simulink model "EcoSIM3_P2_C2_WIP"  (R2014b)
settings: Solver=ode1  SolverMode=SingleTasking  StartTime=0.0  StopTime=4  FixedStep=0.01  RelTol=1e-3
PostLoadFcn:
  | %, if any(exist('dsrtsu_mdlpostloadfcn', 'file') == [2, 3, 6]), try dsrtsu_mdlpostloadfcn('Execute', bdroot); catch fprintf('Error in PostLoadFcn (dsrtsu_mdlpostloadfcn) for model "%s":\n %s\n', bdroot, lasterr); end, end,
InitFcn:
  | tic
  | %Startup_EcoSIM
undefined symbols (not defined in the file or in its folder): canChannel, Controls, DriveCycles, Driver, EM_EFF_MAP, EM_PwrLoss_MAP, EngPwr, EngSpd, EngTrq, Glbl, Overwritten_Mode, Plants, Power, sigbuilder_block, Torque, Trialmap, Veh_Dynamics
libraries: simulink x135, canmsglib x113, fl_lib x104, canlib x89, nesl_utility x56, sdl_lib x29, dspsigops x6, dspswit3 x5, dspstat3 x2, commnoisgen2 x1, dspfdesign x1
(part 1 of 21)
settings Model: DSRTSU_INTERNAL_RTI_VER=450  DSRTSU_INTERNAL_RTI_TYPE=rti1006  RTICANMMDATA=struct('GeneralSetupData',struct('modelroot','C:\Users\EcoCAR_HIL\Documents\Khanna\EcoSIM3_P1_0_PHEV_dynamic_RTI','generalsettings',struct('filesettings',struct('destfolder',struct('Name','RTICANMM_FILES','Check',1),'buildfolder',struct('Name','.','Check',1),'AbsDestfolder',struct('Name','C:\Users\EcoCAR_HIL\Documents\Khanna\EcoSIM3_P1_0_PHEV_dynamic_RTI\RTICANMM_FILES'),'AbsBuildfolder',struct('Name','C:\Users\EcoCAR_HIL\Documents\Khanna\EcoSIM3_P1_0_PHEV_dynamic_RTI'))),'options',struct('addpaths',1,'rmpaths',1,'addtrcexclusion',logical(1),'cannavigator',struct('checkmonitoring',0),'show_usrtrc',0,'use_usrtrc',0),'advanced',struct('options',[1 1 1 1 1 1 1 1 1 1 1 1 1 1 1 1 1 1 1 1 1 1 1 1 1 1 1 1 1 1 1 1 1 1 1 1 1 1 1 1 1 1 1 1 1 1 1 1 1 1 1 1 1 1 1 1 1 1 1 1 1 1 1 1 1 1 1 1 1 1 1 1 1 1 1 1 1 1 1 1 1 1 1 1 1 1 1 1 1 1 1 1 1 1 1 1 1 1 1 1]),'MPSetup',{{}},'modelname','EcoSIM3_P1_0_PHEV_2014b_with_inertia','block','EcoSIM3_P1_0_PHEV_2014b_with_inertia'))  DSRTSU_INTERNAL_RTIFPGA=40  CovPath=GCM/ProcessMode  CovHTMLOptions=-sRT=1 -sVT=0 -aTS=1 -bRG=1 -bTC=1 -hTR=0 -nFC=0 -scm=1 -bcm=1 -xEv=0  Creator=Arjun  LastModifiedBy=Aditya
settings ConfigSet: Description=This configuration is meant for HIL simulations. During HIL simulations, the model should use dSPACE's rti1006 to generate code.
settings DataIOCC: InspectSignalLogs=on
settings OptimizationCC: BlockReduction=off
settings DebuggingCC: UnderspecifiedInitializationDetection=Classic  MergeDetectMultiDrivingBlocksExec=none  MultiTaskCondExecSysMsg=warning
settings HardwareCC: ProdIntDivRoundTo=Zero  ProdEndianess=LittleEndian  ProdHWDeviceType=Generic->Custom  TargetIntDivRoundTo=Zero  TargetEndianess=LittleEndian  TargetHWDeviceType=Generic->Custom
settings RTWCC: SystemTargetFile=rti1006.tlc  MakeCommand=make_rti  TemplateMakefile=rti1006.tmf  Description=dSPACE DS1006 Hardware Platform  ProcessScript=rti1006_make_rtw_hook
settings STFCustomTargetCC: ParMdlRefBuildCompliant=on  GeneratePreprocessorConditionals=Disable all  SystemTargetFile=rti1006.tlc
settings GRTTargetCC: CompOptLevelCompliant=off  ConcurrentExecutionCompliant=off  CombineOutputUpdateFcns=off  MatFileLogging=off  CPPClassGenCompliant=off  GRTInterface=on  ExtModeMexFile=noextcomm
settings SimscapeCC: SelectedTab=Simscape

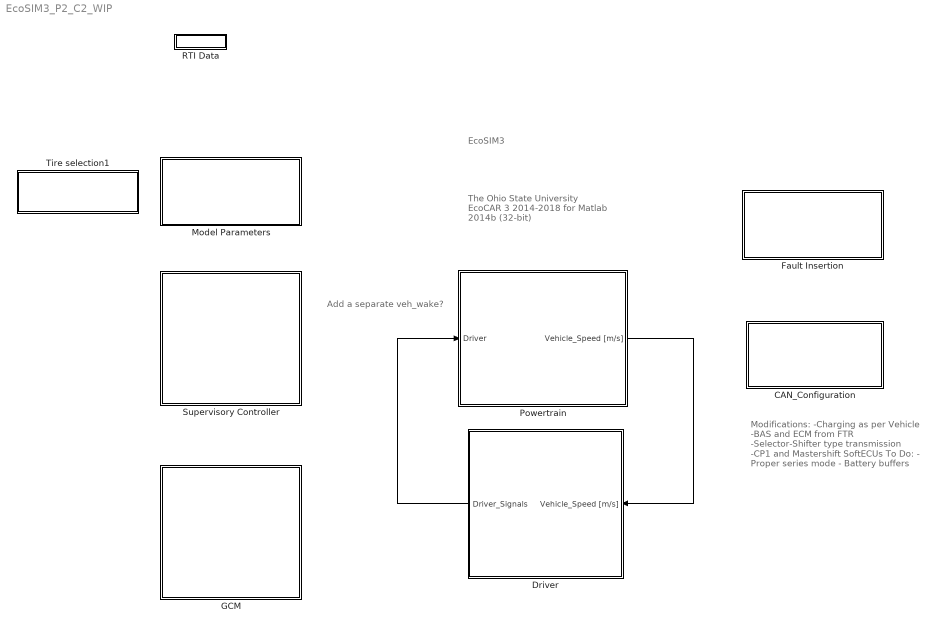
== system EcoSIM3_P2_C2_WIP ==
  note: Add a separate veh_wake?
  note: Modifications:
      | -Charging as per Vehicle
      | -BAS and ECM from FTR
      | -Selector-Shifter type transmission
      | -CP1 and Mastershift SoftECUs
      |
      | To Do:
      | - Proper series mode
      | - Battery buffers
  note: The Ohio State University
      | EcoCAR 3 2014-2018
      | for Matlab 2014b (32-bit)
  note: EcoSIM3
  CAN_Configuration : Subsystem  Variant=on  VariantControl=Sim_type == 1
  Driver : Subsystem
      mask Display: image(imread('images/BRUTUS.png'))
  Fault Insertion : Subsystem
  GCM : Subsystem  SystemSampleTime=0.001  VariantControl=Variant1
      settings: MinAlgLoopOccurrences=on
      mask Display: image(imread('images/GCM.jpg'))
  Model Parameters : Subsystem  mask{DRIV_cycle=US06 - Highway portion, DRIV_mode=Normal, Propulsion_mode=Individual, Simulation_mode=Velocity Profile, Grade=0, Init_SOC=50, Veh_Plugged_In=off}
      mask prompts: DRIV_cycle "Drive Cycle"; DRIV_mode "Drive Mode"; Propulsion_mode "Propulsion"; Simulation_mode "Simulation Mode"; Grade "Grade [%]"; Init_SOC "Initial SOC [%]"; Veh_Plugged_In "Charging Mode"
      mask help: Model Parameters Available for Modification
      mask TypeOptions DRIV_cycle: FUDS | FHDS | US06 | UDDS - 505 portion | US06 - City portion | US06 - Highway portion | Gradeability Test | Acceleration Test | Demo Cycle | Y3 Fall Report Cycle
      mask TypeOptions DRIV_mode: Normal | Performance
      mask TypeOptions Propulsion_mode: Individual | Blended
      mask TypeOptions Simulation_mode: Velocity Profile | Comparison
      mask Display: disp('Simulation\nParameters')
  Powertrain : Subsystem
      mask Display: image(imread('images/OSU_EC3_Powertrain.png'))
  RTI Data : Subsystem  Tag=struct('RTIDataServer',struct('RTIDataServerVs','2','RTIModelDescription','struct(''main'',''EcoSIM3_P2_C2_WIP'',''sub'',''EcoSIM3_P2_C2_WIP'',''isMp'',0)'))  LoadFcn="if exist('rtidc'), try,  rtidc('DataHostBlockClbLoad', gcbh); catch, disp(['Warning: ''LoadFcn'' for RTI Data block failed: ' lasterr]); end, end,"  mask(RTI_DATA_HOST){}
      mask help:
      | RTI Data Block.
      | This block is used by RTI to store internal model-dependent data.
      | Please keep this block on the root level of the model. Deleting this block will result in data loss.
      |
      | NEVER DELETE OR COPY THIS BLOCK!
      settings: CopyFcn="if exist('rtidc'), try,  rtidc('DataHostBlockClbCopy', gcbh); catch, disp(['Warning: ''CopyFcn'' for RTI Data block failed: ' lasterr]); end, end,"  DeleteFcn="if exist('rtidc'), try,  rtidc('DataHostBlockClbDelete', gcbh); catch, disp(['Warning: ''DeleteFcn'' for RTI Data block failed: ' lasterr]); end, end,"  ModelCloseFcn="if exist('rtidc'), try,  rtidc('DataHostBlockClbModelClose', gcbh); catch, disp(['Warning: ''ModelCloseFcn'' for RTI Data block failed: ' lasterr]); end, end,"  PreSaveFcn="if exist('rtidc'), try,  rtidc('DataHostBlockClbPreSave', gcbh); catch, disp(['Warning: ''PreSaveFcn'' for RTI Data block failed: ' lasterr]); end, end,"  PostSaveFcn="if exist('rtidc'), try,  rtidc('DataHostBlockClbPostSave', gcbh); catch, disp(['Warning: ''PostSaveFcn'' for RTI Data block failed: ' lasterr]); end, end,"  NameChangeFcn="if exist('rtidc'), try,  rtidc('DataHostBlockClbNameChange', gcbh); catch, disp(['Warning: ''NameChangeFcn'' for RTI Data block failed: ' lasterr]); end, end,"
      mask Help:
      | RTI Data Block.
      | This block is used by RTI to store internal model-dependent data.
      | Please keep this block on the root level of the model. Deleting this block will result in data loss.
      | 
      | NEVER DELETE OR COPY THIS BLOCK!
      mask Display:
      | text(0.5, 0.5, 'RTI Data', 'HorizontalAlignment', 'center');
      | plot([1 0]);
  Supervisory Controller : Subsystem  SystemSampleTime=0.001  VariantControl=Variant1
      settings: MinAlgLoopOccurrences=on
      mask Display: image(imread('images/super.jpg'))
  Tire selection1 : Subsystem  mask{dynodata=AccelerationTest250Nm}
      mask prompts: dynodata "Dyno Data"
      mask help: Dtermine which drive cycle from dyno is used for comparison
      mask init:
      | if strcmp(dynodata,'AccelerationTest250Nm')
      |     evalin('base','dynocycle = 1;');
      |     evalin('base','load AcclnTest250');
      | elseif strcmp(dynodata,'US06_150Nm')
      |     evalin('base','dynocycle = 2;');
      |     evalin('base','load US06_150');
      | elseif strcmp(dynodata,'Coastdown')
      |     evalin('base','dynocycle = 3;');
      |     evalin('base','load Coastdown');
      | elseif strcmp(dynodata,'HWFET_150Nm')
      |     evalin('base','dynocycle = 4;');
      |     evalin('base','load HWFET_150');
      | end
      mask TypeOptions dynodata: AccelerationTest250Nm | US06_150Nm | Coastdown | HWFET_150Nm
      mask Display:
      | fprintf('Comparison Data:\n\n')
      | fprintf(dynodata);
  wires:
  Powertrain/1(Vehicle_Speed [m/s]) -> Driver/1(Vehicle_Speed [m/s])
  Driver/1(Driver_Signals) -> Powertrain/1(Driver)

== system EcoSIM3_P2_C2_WIP/CAN_Configuration ==
  From_Goto : Subsystem  VariantControl=Sim_type == 1
  MIL_SIL_Kvaser : Subsystem  VariantControl=Sim_type == 3
  MIL_SIL_Vector : Subsystem  VariantControl=Sim_type == 2

== system EcoSIM3_P2_C2_WIP/Driver ==
  note: Driver
  Vehicle_Speed [m/s] : Inport
  APP : Subsystem
  Bias : Bias  Bias=-1
  Bus Creator : BusCreator  Inputs=7
  Bus Selector : BusSelector  OutputSignals=Simulation_mode,Velocity_Profile_m_per_s,Veh_Plugged_In
  Bus Selector1 : BusSelector  OutputSignals=Vehicle_Speed_meter_per_s
  Constant : Constant  Commented=on  Value=0
  Drive_Mode : Constant
  GM_Transmit : Subsystem
  PI Controller : Subsystem
  PRND Elec : Subsystem
  PRNDL : Constant  Commented=on
  PRNDL_Input : Step  Time=1.8  Before=1  After=4  SampleTime=0
  Ramp : simulink/Sources/Ramp  Commented=on  slope=1  start=0  X0=-1
  Rounding Function : Rounding  Commented=on
  Saturation : Saturate  Commented=on  UpperLimit=4  LowerLimit=1
  Scope : Scope  NumInputPorts=2
      settings: YMin=-5~-5  YMax=5~5  SaveName=ScopeData57
  Startup Dummy : Subsystem
  Step : Step  Time=5  After=30  SampleTime=0
  Switch : Switch  Criteria=u2 > Threshold  Threshold=0.5
  Driver_Signals : Outport
  wires:
  PI Controller/1(Alpha [%]) -> APP/1(Pos_AccPedal[%])
  [Simulation_Parameters] -> Bus Selector/1
  PRNDL_Input/1 -> PRND Elec/1(PRNDL), Startup Dummy/1(PRNDL), Bus Creator/4  "PRNDL"
  PI Controller/2(Beta [%]) -> Startup Dummy/2(Beta)
  Vehicle_Speed [m/s]/1 -> GM_Transmit/3(CAN2), Bus Selector1/1
  Bus Selector1/1 -> Scope/2, PI Controller/2(Vehicle_Speed [m/s]), Startup Dummy/4(VehSpeed)  "<Vehicle_Speed_meter_per_s>"
  Drive_Mode/1 -> Bus Creator/1  "Drive_Mode"
  APP/1(Accel_Low[V]) -> Bus Creator/5
  APP/2(Accel_High[V]) -> Bus Creator/6
  Startup Dummy/1(KeyState) -> Bus Creator/7
  GM_Transmit/1(Driver_Signals) -> Driver_Signals/1
  Bus Creator/1 -> GM_Transmit/1(Electrical)
  Startup Dummy/2(Vehicle Out) -> GM_Transmit/2(CAN1)
  Bus Selector/3 -> Startup Dummy/3(PluggedIn)  "<Veh_Plugged_In>"
  Ramp/1 -> Rounding Function/1
  Rounding Function/1 -> Saturation/1
  PRND Elec/1(PRNDL1[V]) -> Bus Creator/2
  PRND Elec/2(PRNDL2[V]) -> Bus Creator/3
  Bias/1 -> Switch/2
  Bus Selector/1 -> Bias/1  "<Simulation_mode>"
  Switch/1 -> Scope/1, PI Controller/1(Velocity_Profile [m/s])  "Velocity_Profile_m_per_s"
  [DynoSpeed] -> Switch/1
  Step/1 -> Switch/3

== system EcoSIM3_P2_C2_WIP/Fault Insertion ==
  EM_Inverter_Triggers : Subsystem
  ESS Triggers : Subsystem

== system EcoSIM3_P2_C2_WIP/GCM ==
  note: Do we have to use the supervisory wakeup signal in MIL?
      | We could put the RTI DIG block in the GCM built model to
      | power up the supervisory
  Bus Creator2 : BusCreator  Inputs=2
  GCM_IO : Subsystem  Variant=on
  ProcessMode : Subsystem
  tag scope: GCM_To_CAN=global
  wires:
  [GCM_from_CAN] -> ProcessMode/1(In1)
  Bus Creator2/1 -> [GCM_To_CAN]  "GCM_Transmit"
  ProcessMode/2(RelaySignals) -> Bus Creator2/2  "GCM_Electrical_Out"
  ProcessMode/1(CAN) -> Bus Creator2/1

== system EcoSIM3_P2_C2_WIP/Model Parameters ==
  Bias : Bias  Bias=-1
  Bus Creator : BusCreator  Inputs=6
  Clock : Clock
  Cycle Length : Subsystem
  Drive Cycle : Constant  Value=DRIV_cycle
  Drive Cycle Selection : Subsystem
  Initial_SOC : Constant  Value=Init_SOC
  Input : Constant  Value=Simulation_mode
  Input1 : Constant  Value=Simulation_mode
  Mode : Constant  Value=DRIV_mode
  Plugged_In : Constant  Value=Veh_Plugged_In
  Propulsion : Constant  Value=Propulsion_mode
  Relational Operator2 : RelationalOperator  InputSameDT=on
  Stop Simulation : Stop
  Switch : Switch  Criteria=u2 > Threshold  Threshold=0.5
  Switch1 : Switch  Criteria=u2 > Threshold  Threshold=0.5
  tag scope: Simulation_Parameters=global
  wires:
  Bus Creator/1 -> [Simulation_Parameters]  "Simulation_Parameters"
  Switch/1 -> Stop Simulation/1
  Clock/1 -> Relational Operator2/1  "sim_time"
  Initial_SOC/1 -> Bus Creator/3  "Init_SOC_percent"
  Drive Cycle Selection/1(Cycle Velocity) -> Bus Creator/2
  Drive Cycle/1 -> Drive Cycle Selection/1(Drive Cyc Selection), Cycle Length/1(Drive Cyc Selection)
  Plugged_In/1 -> Switch/2, Bus Creator/1  "Veh_Plugged_In"
  Relational Operator2/1 -> Switch/3
  [Charging_Complete] -> Switch/1
  Mode/1 -> Bus Creator/4  "DRIV_mode"
  Propulsion/1 -> Bus Creator/5  "Propulsion_mode"
  Input/1 -> Bus Creator/6  "Simulation_mode"
  Cycle Length/1(Cycle Time) -> Switch1/3
  [CycleTime] -> Switch1/1
  Switch1/1 -> Relational Operator2/2
  Bias/1 -> Switch1/2
  Input1/1 -> Bias/1

== system EcoSIM3_P2_C2_WIP/Powertrain ==
  note: Powertrain
  Driver : Inport
  Accessories Power Module : Subsystem
      mask Display: image(imread('images/DCDC_iso.png'))
  BAS Motor : Subsystem
      mask Display: image(imread('images/BAS.png'))
  Belt Coupler : Subsystem
      mask Display: image(imread('images/belt.png'))
  Bus Selector : BusSelector  OutputSignals=GMLAN_CAN_Out.PPEI_Brake_Apply_Status.BrkPdlPos
  Charger : Subsystem
      mask Display: image(imread('images/brusa.png'))
  Clutch_Transmission1 : Subsystem  Commented=on
  Clutch_Transmission2 : Subsystem
      mask Display: image(imread('images/Trans.png'))
  "Electric Motor " : Subsystem
      mask Display: image(imread('images/EM.png'))
  Electrical Storage System : Subsystem
      mask Display: image(imread('images/ESS.png'))
  Engine : Subsystem
      mask Display: image(imread('images/Engine.png'))
  Fuel Tank : Subsystem
      mask Display: image(imread('images/Fuel_Tank.png'))
  Mechanical Coupler : Subsystem
      mask Display: image(imread('images/PTU.png'))
  Soft_ECUs_IO : Subsystem  Variant=on
  Vehicle Dynamics : Subsystem
      mask Display: image(imread('images/2016camaro.png'))
  Vehicle_Speed [m/s] : Outport
  tag scope: GM_Transmit=global
  wires:
  Accessories Power Module/1(Accessories_Power_In_W) -> Electrical Storage System/2(Accessories_Power_In [W])
  "Electric Motor "/1(To_Battery) -> Electrical Storage System/3(EM_Power_In [W])
  BAS Motor/1(BAS_Power_in [W]) -> Electrical Storage System/4(BAS_Power_In [W])
  Engine/1(Fuel_Consumption) -> Fuel Tank/1(ICE_m_f_dot [kg/s])
  Vehicle Dynamics/1(Vehicle_Speed [m/s]) -> Vehicle_Speed [m/s]/1
  Bus Selector/1 -> Vehicle Dynamics/1(Beta)  "<BrkPdlPos>"
  Driver/1 -> [GM_Transmit], Bus Selector/1
  Charger/1(Charger_Power_W) -> Electrical Storage System/1(Charger_Power_In [W])
  connections:
  Engine/RConn1 -- Belt Coupler/LConn2
  Mechanical Coupler/RConn1 -- Vehicle Dynamics/LConn1
  "Electric Motor "/RConn1 -- Mechanical Coupler/LConn1
  Mechanical Coupler/LConn2 -- Clutch_Transmission2/RConn1
  Belt Coupler/RConn1 -- Clutch_Transmission2/LConn1
  BAS Motor/RConn1 -- Belt Coupler/LConn1

== system EcoSIM3_P2_C2_WIP/RTI Data ==
  RTI Data Store : Subsystem  Tag=struct('private',struct('version',struct('dsVer',uint32(2)),'access',struct('modified',['07-Jul-2016 12:18:38'],'type','Model','isPerm',1)),'public',struct('main',struct('data',[]),'sub',struct('name','','data',[])))  mask(RTI_DATA_STORE){}
      mask help:
      | RTI Data Store Block. This block is used by RTI to store internal model dependent data. Deleting this block will result in data loss.
      |
      | NEVER DELETE, COPY, OR MODIFY THIS BLOCK!
      mask Help:
      | RTI Data Store Block. This block is used by RTI to store internal model dependent data. Deleting this block will result in data loss.
      | 
      | NEVER DELETE, COPY, OR MODIFY THIS BLOCK!
      mask Display: text(0.5, 0.5, ' ', 'HorizontalAlignment', 'center');

== system EcoSIM3_P2_C2_WIP/Supervisory Controller ==
  Bus Creator1 : BusCreator  Inputs=2
  Charging Handshake : Subsystem
  Clutch Request : Subsystem
  Display : Display
  Driver Requested Torque : Subsystem
  Functional Safety1 : Subsystem  Commented=on
  Input Conditioning : Subsystem
  Mode Operation : Subsystem
  "Mode Selection " : Subsystem
  Outout Conditioning : Subsystem
  PRNDL : Subsystem
  Simple Fault Detection : Subsystem
  Subsystem : Subsystem
  Supervisory_IO : Subsystem  Variant=on
  tag scope: Mode=global, To_Vehicle=global
  wires:
  [From_Vehicle] -> Input Conditioning/1(Raw Signals), Charging Handshake/1(In1), Simple Fault Detection/1(In1)
  "Mode Selection "/1(Mode Transmit) -> Display/1, [Mode], Bus Creator1/2  "Mode"
  Driver Requested Torque/1(Driver Torque Request) -> Bus Creator1/1
  Simple Fault Detection/1("Fault Code ") -> "Mode Selection "/2("Fault_Code ")
  Bus Creator1/1 -> Mode Operation/1(Supervisory)
  Input Conditioning/1(Conditioned Signals) -> PRNDL/2("From CAN "), Clutch Request/2(CAN), Subsystem/1(In1), Mode Operation/2(From CAN), "Mode Selection "/1(CAN IN), Driver Requested Torque/1(CAN IN)
  PRNDL/1("Total Torque ") -> Outout Conditioning/2(In1)
  Mode Operation/1(Component Torque Request) -> "Mode Selection "/3(Startup), Clutch Request/1(Component Req), PRNDL/1(Controller Inputs)
  Outout Conditioning/1(Out1) -> [To_Vehicle]
  Charging Handshake/1(Out1) -> Outout Conditioning/4(In2)
  Clutch Request/1(Out1) -> PRNDL/3(Clutch), Outout Conditioning/3(CP1)
  Subsystem/1(Out1) -> Outout Conditioning/1(NonProp)

== system EcoSIM3_P2_C2_WIP/Tire selection1 ==

== system EcoSIM3_P2_C2_WIP/CAN_Configuration/From_Goto ==
  Ground : Ground
  Terminator : Terminator
  wires:
  Ground/1 -> Terminator/1

== system EcoSIM3_P2_C2_WIP/CAN_Configuration/MIL_SIL_Kvaser ==
  CAN Configuration : canlib/CAN Configuration  BlockHandle=18.0005  DeviceMenu=Kvaser Virtual 1 (Channel 1)  Device=Kvaser Virtual 1 (Channel 1)  ObjConstructor=canChannel('Kvaser', 'Virtual 1', 1)  BusSpeed=500000  EnableBitParameters=off  SJW=1  TSEG1=4  TSEG2=3  NSamples=1  AckMode=Normal
  CAN Configuration1 : canlib/CAN Configuration  BlockHandle=19.0005  DeviceMenu=Kvaser Virtual 1 (Channel 2)  Device=Kvaser Virtual 1 (Channel 2)  ObjConstructor=canChannel('Kvaser', 'Virtual 1', 2)  BusSpeed=500000  EnableBitParameters=off  SJW=1  TSEG1=4  TSEG2=3  NSamples=1  AckMode=Normal

== system EcoSIM3_P2_C2_WIP/CAN_Configuration/MIL_SIL_Vector ==
  CAN Configuration : canlib/CAN Configuration  BlockHandle=5560.0004  DeviceMenu=Vector Virtual 1 (Channel 1)  Device=Vector Virtual 1 (Channel 1)  ObjConstructor=canChannel('Vector', 'Virtual 1', 1)  BusSpeed=500000  EnableBitParameters=off  SJW=1  TSEG1=4  TSEG2=3  NSamples=1  AckMode=Normal
  CAN Configuration1 : canlib/CAN Configuration  BlockHandle=5561.0004  DeviceMenu=Vector Virtual 1 (Channel 2)  Device=Vector Virtual 1 (Channel 2)  ObjConstructor=canChannel('Vector', 'Virtual 1', 2)  BusSpeed=500000  EnableBitParameters=off  SJW=1  TSEG1=4  TSEG2=3  NSamples=1  AckMode=Normal

== system EcoSIM3_P2_C2_WIP/Driver/APP ==
  Pos_AccPedal[%] : Inport
  Add : Sum  Commented=on
  Constant : Constant  Value=.4
  Constant1 : Constant  Value=.8
  Constant2 : Constant  Commented=on  Value=.4
  Constant3 : Constant  Commented=on  Value=.8
  Constant4 : Constant  Commented=on  Value=40
  Constant5 : Constant  Commented=on  Value=.4
  Constant6 : Constant  Commented=on  Value=.8
  Display : Display  Commented=on
  Gain_APM1 : Gain  Gain=0.0021
  Offset_APM1 : Constant  Value=0.009
  Output Scaling1 : Gain  Gain=1/50
  Output Scaling2 : Gain  Gain=1/25
  Output Scaling3 : Gain  Commented=on  Gain=1/50
  Output Scaling4 : Gain  Commented=on  Gain=1/25
  Output Scaling5 : Gain  Commented=on  Gain=50
  Output Scaling6 : Gain  Commented=on  Gain=25
  Output Scaling7 : Gain  Commented=on  Gain=0.5
  Sum : Sum  Inputs=++|
  Sum1 : Sum  Inputs=|++
  Sum2 : Sum  Commented=on  Inputs=++|
  Sum3 : Sum  Commented=on  Inputs=|++
  Sum4 : Sum  Commented=on  Inputs=-+|
  Sum5 : Sum  Commented=on  Inputs=|+-
  Sum6 : Sum  Inputs=++|
  Accel_Low[V] : Outport
  Accel_High[V] : Outport  Port=2
  wires:
  Constant/1 -> Sum/1
  Sum/1 -> Accel_Low[V]/1  "Alpha_Low"
  Output Scaling1/1 -> Sum/2
  Pos_AccPedal[%]/1 -> Output Scaling2/1, Output Scaling1/1
  Constant1/1 -> Sum1/2
  Output Scaling2/1 -> Sum1/1
  Sum1/1 -> Accel_High[V]/1  "Alpha_High"
  Constant2/1 -> Sum2/1
  Sum2/1 -> Sum4/2  "Alpha_Low"
  Output Scaling3/1 -> Sum2/2
  Constant4/1 -> Output Scaling4/1, Output Scaling3/1
  Constant3/1 -> Sum3/2
  Output Scaling4/1 -> Sum3/1
  Sum3/1 -> Sum5/1  "Alpha_High"
  Constant5/1 -> Sum4/1
  Constant6/1 -> Sum5/2
  Sum4/1 -> Output Scaling5/1
  Sum5/1 -> Output Scaling6/1
  Output Scaling5/1 -> Add/1
  Output Scaling6/1 -> Add/2
  Add/1 -> Output Scaling7/1
  Output Scaling7/1 -> Display/1
  Sum6/1 -> ?  "Alpha_Low"
  ? -> Gain_APM1/1
  Gain_APM1/1 -> Sum6/2
  Offset_APM1/1 -> Sum6/1

== system EcoSIM3_P2_C2_WIP/Driver/GM_Transmit ==
  Electrical : Inport
  CAN1 : Inport  Port=2
  CAN2 : Inport  Port=3
  Bus Creator : BusCreator  Inputs=2
  Bus Creator1 : BusCreator  Inputs=7
  Bus Creator2 : BusCreator  Inputs=5
  Bus Creator3 : BusCreator  Inputs=2
  Bus Creator4 : BusCreator  Inputs=2
  Bus Creator5 : BusCreator  Inputs=1
  Bus Creator6 : BusCreator  Inputs=1
  Bus Creator7 : BusCreator  Inputs=1
  Bus Selector : BusSelector  OutputSignals=Drive_Mode,PRNDL,Alpha_Low,Alpha_High,Accessory_Wake,PRNDL_1,PRNDL_2
  Bus Selector1 : BusSelector  OutputSignals=SysPwrMd,BrkPdlPos,Vehicle_Speed_meter_per_s
  Bus Selector2 : BusSelector  OutputSignals=Rear_Right_Tire_Angle,Rear_Left_Tire_Angle,Front_Right_Tire_Angle,Front_Left_Tire_Angle
  Display : Display
  Gain : Gain  Gain=3.6
  Gain1 : Gain
  WheelTickLD : Subsystem
  WheelTickLND : Subsystem
  WheelTickRD : Subsystem
  WheelTickRND : Subsystem
  Driver_Signals : Outport
  wires:
  Bus Creator4/1 -> Bus Creator2/5  "PPEI_NonDrivn_Whl_Rotationl_Stat"
  CAN1/1 -> Bus Selector1/1
  Bus Creator1/1 -> Bus Creator/1  "GM_Electrical_Out"
  Bus Creator3/1 -> Bus Creator2/4  "PPEI_Driven_Whl_Rotational_Stat"
  Electrical/1 -> Bus Selector/1
  Bus Creator/1 -> Driver_Signals/1  "GM_Transmit"
  Bus Creator2/1 -> Bus Creator/2  "GMLAN_CAN_Out"
  Bus Selector/1 -> Bus Creator1/1  "<Drive_Mode>"
  Bus Selector/2 -> Bus Creator1/2  "<PRNDL>"
  Bus Selector/3 -> Bus Creator1/3  "<Alpha_Low>"
  Bus Selector/4 -> Bus Creator1/4  "<Alpha_High>"
  Bus Selector/5 -> Bus Creator1/5  "<Accessory_Wake>"
  Bus Creator5/1 -> Bus Creator2/2  "PPEI_Brake_Apply_Status"
  Bus Selector1/1 -> Gain1/1  "<SysPwrMd>"
  Bus Creator6/1 -> Bus Creator2/1  "PPEI_Platform_General_Status"
  Bus Selector1/3 -> Gain/1  "<Vehicle_Speed_meter_per_s>"
  Gain/1 -> Bus Creator7/1  "VehSpdAvgDrvn"
  Bus Creator7/1 -> Bus Creator2/3  "PPEI_Vehicle_Speed_and_Distance"
  CAN2/1 -> Bus Selector2/1
  Bus Selector2/4 -> WheelTickLND/1(In1)  "<Front_Left_Tire_Angle>"
  Bus Selector2/2 -> WheelTickLD/1(In1)  "<Rear_Left_Tire_Angle>"
  Bus Selector2/3 -> WheelTickRND/1(In1)  "<Front_Right_Tire_Angle>"
  Bus Selector2/1 -> WheelTickRD/1(In1)  "<Rear_Right_Tire_Angle>"
  Bus Selector1/2 -> Bus Creator5/1  "<BrkPdlPos>"
  Gain1/1 -> Display/1, Bus Creator6/1  "SysPwrMd"
  WheelTickRD/1(Out1) -> Bus Creator3/1
  WheelTickLD/1(Out1) -> Bus Creator3/2
  WheelTickRND/1(Out1) -> Bus Creator4/1
  WheelTickLND/1(Out1) -> Bus Creator4/2
  Bus Selector/6 -> Bus Creator1/6  "<PRNDL_1>"
  Bus Selector/7 -> Bus Creator1/7  "<PRNDL_2>"

== system EcoSIM3_P2_C2_WIP/Driver/PI Controller ==
  note: The accelerator override is used to press the ac pedal to check ac pedal startup requirement.
  Velocity_Profile [m/s] : Inport
  Vehicle_Speed [m/s] : Inport  Port=2
  Bias : Bias  Bias=-1
  Brake_Override : Constant  Commented=on  Value=0
  Bus Selector : BusSelector  OutputSignals=Shift_In_Progress
  Bus Selector1 : BusSelector  OutputSignals=Simulation_mode
  Compare To Zero1 : simulink/Logic and Bit Operations/Compare To Zero  relop===  OutDataTypeStr=boolean  ZeroCross=off
  Delay : Subsystem
  Dyno Data Variant : Subsystem  Variant=on
  I : Constant  Value=Driver.I
  Integrator1 : Integrator  ExternalReset=level
  Memory : Memory
  Memory1 : Memory
  P : Constant  Value=Driver.P
  Percent_beta : Constant  Value=10
  Product3 : Product  RndMeth=Zero
  Product4 : Product  RndMeth=Zero
  Saturation (-1 to 0)1 : Saturate  UpperLimit=0  LowerLimit=-100
  Saturation (0 to 1)1 : Saturate  UpperLimit=100  LowerLimit=0
  Scope : Scope
      settings: SaveName=ScopeData8
  Scope1 : Scope
      settings: SaveName=ScopeData54
  Scope2 : Scope
      settings: SaveName=ScopeData55
  Sum3 : Sum  Inputs=|-+  SaturateOnIntegerOverflow=on  InputSameDT=on  OutDataTypeStr=Inherit: Same as first input
  Sum4 : Sum  SaturateOnIntegerOverflow=on  InputSameDT=on  OutDataTypeStr=Inherit: Same as first input
  Sum5 : Sum  Inputs=|+-  SaturateOnIntegerOverflow=on  InputSameDT=on  OutDataTypeStr=Inherit: Same as first input
  Switch : Switch  Criteria=u2 > Threshold  Threshold=0.5
  Switch1 : Switch  Criteria=u2 > Threshold  Threshold=0.5
  Switch2 : Switch  Criteria=u2 > Threshold  Threshold=0.5
  gain1 : Gain  Gain=-1  SaturateOnIntegerOverflow=on  OutDataTypeStr=Inherit: Same as input  ParamDataTypeStr=Inherit: Same as input
  Alpha [%] : Outport
  Beta [%] : Outport  Port=2
  wires:
  Saturation (-1 to 0)1/1 -> gain1/1
  Sum4/1 -> Saturation (0 to 1)1/1, Saturation (-1 to 0)1/1
  Vehicle_Speed [m/s]/1 -> Sum3/1, Compare To Zero1/1, Sum5/2
  Product4/1 -> Sum4/1
  Product3/1 -> Sum4/2
  Compare To Zero1/1 -> Integrator1/2
  Integrator1/1 -> Product3/1
  Velocity_Profile [m/s]/1 -> Scope2/1, Sum5/1, Delay/1(Velocity_Profile [m/s])
  Sum5/1 -> Product4/2
  Switch/1 -> Memory/1, Alpha [%]/1, Switch2/3  "Alpha_percentage"
  Delay/1(Pre_Velocity_Profile [m/s]) -> Sum3/2
  Sum3/1 -> Integrator1/1
  I/1 -> Product3/2
  P/1 -> Product4/1
  gain1/1 -> Scope/1, Beta [%]/1  "Beta_percentage"
  Percent_beta/1 -> Switch1/3  "Beta_percentage"
  Memory/1 -> Switch2/1
  [Driver_SoftECU_Receive] -> Bus Selector/1
  Bus Selector/1 -> Scope1/1, Memory1/1  "<Shift_In_Progress>"
  Memory1/1 -> Switch2/2
  Saturation (0 to 1)1/1 -> Switch/3
  [Simulation_Parameters] -> Bus Selector1/1
  Bus Selector1/1 -> Bias/1  "<Simulation_mode>"
  Bias/1 -> Switch/2
  Dyno Data Variant/1(Alpha) -> Switch/1

== system EcoSIM3_P2_C2_WIP/Driver/PRND Elec ==
  PRNDL : Inport
  Constant : Constant  Value=0.65
  Constant1 : Constant  Value=1.30
  Constant2 : Constant  Value=1.65
  Constant3 : Constant  Value=2.0
  Constant4 : Constant  Value=0.45
  Constant5 : Constant  Value=1.1
  Constant6 : Constant  Value=1.5
  Constant7 : Constant  Value=1.8
  Gain : Gain  Gain=0.1
  Gain1 : Gain  Gain=0.1
  Multiport Switch : MultiPortSwitch  Inputs=4
  Multiport Switch1 : MultiPortSwitch  Inputs=4
  PRNDL1[V] : Outport
  PRNDL2[V] : Outport  Port=2
  wires:
  PRNDL/1 -> Multiport Switch1/1, Multiport Switch/1
  Constant/1 -> Multiport Switch/2
  Constant1/1 -> Multiport Switch/3
  Constant2/1 -> Multiport Switch/4
  Constant3/1 -> Multiport Switch/5
  Constant4/1 -> Multiport Switch1/2
  Constant5/1 -> Multiport Switch1/3
  Constant6/1 -> Multiport Switch1/4
  Constant7/1 -> Multiport Switch1/5
  Gain/1 -> PRNDL1[V]/1  "PRNDL_1"
  Gain1/1 -> PRNDL2[V]/1  "PRNDL_2"
  Multiport Switch/1 -> Gain/1  "PRNDL_1"
  Multiport Switch1/1 -> Gain1/1  "PRNDL_2"

== system EcoSIM3_P2_C2_WIP/Driver/Startup Dummy ==
  note: Key_Sw is the electrical signal to wake the GCM. It is triggered by either
      | the push button or plugging the Brusa in.
  note: VehStart is a processed signal to emulate SysPwrMd in GMLAN
  PRNDL : Inport
  Beta : Inport  Port=2
  PluggedIn : Inport  Port=3
  VehSpeed : Inport  Port=4
  Bus Creator : BusCreator  Inputs=3
  Bus Selector : BusSelector  OutputSignals=Brusa_Electrical_Out.GCM_Wakeup_charge
  Chart : Stateflow chart  TreatAsAtomicUnit=on
  Constant : Constant  Value=0
  Logical Operator : Logic  Operator=OR  AllPortsSameDT=off  OutDataTypeStr=boolean
  PulseStart : DiscretePulseGenerator  Commented=on  PulseType=Time based  Period=3  PulseWidth=10
  Start Button : Step  Before=1  After=0  SampleTime=0
  Switch : Switch  Criteria=u2 > Threshold  Threshold=0.5
  Terminator : Terminator
  Vehicle Start : Subsystem
  KeyState : Outport
  Vehicle Out : Outport  Port=2
  wires:
  Switch/1 -> Chart/1(input), Vehicle Start/2(Key Pos)  "Key_State"
  Logical Operator/1 -> Terminator/1  "Key_Sw"
  [Brusa_SoftECU_Transmit] -> Bus Selector/1
  Vehicle Start/2(SysPwrMd) -> Bus Creator/1  "SysPwrMd"
  Beta/1 -> Vehicle Start/3(Brake_Position)
  Vehicle Start/3(Brake Position) -> Bus Creator/2
  Bus Creator/1 -> Vehicle Out/1  "CAN"
  VehSpeed/1 -> Bus Creator/3
  Bus Selector/1 -> Logical Operator/2  "<GCM_Wakeup_charge>"
  Vehicle Start/1(Key State) -> KeyState/1
  Chart/1(output) -> Logical Operator/1
  PRNDL/1 -> Vehicle Start/1(PRNDL)
  PluggedIn/1 -> Switch/2
  Start Button/1 -> Switch/3  "Key_State"
  Constant/1 -> Switch/1

== system EcoSIM3_P2_C2_WIP/Fault Insertion/EM_Inverter_Triggers ==
  Bus Creator{,1..2,4} (4 alike) : BusCreator  Inputs=2
  EM_Faulty_Temperature : Constant  Value=0
  EM_Inverter_Faulty_Temperature : Constant  Value=0
  EM_torque_cmd_rigger : Step  Time=18  After=0  SampleTime=0
  EM_torque_cmd_value : Constant  Value=0
  Step : Step  Time=18  After=0  SampleTime=0
  Trigger : Step  Time=18  After=0  SampleTime=0
  Trigger1 : Step  Time=18  After=0  SampleTime=0
  vsm_state_trigger : Step  Time=18  After=0  SampleTime=0
  vsm_state_value : Constant  Value=0
  tag scope: EM_Inverter_Over_temperature_Trigger=global, EM_OverTorque_Trigger=global, EM_Over_temperature_Trigger=global, EM_Torque_Cmd_Trigger=global, VSM_State_Trigger=global
  wires:
  Bus Creator4/1 -> [VSM_State_Trigger]  "vsm_state_fault"
  vsm_state_trigger/1 -> Bus Creator4/1  "vsm_state_trigger"
  vsm_state_value/1 -> Bus Creator4/2  "vsm_state_value"
  Trigger/1 -> Bus Creator/1  "EM_OverTemp_Trigger"
  Step/1 -> [EM_OverTorque_Trigger]  "EM_OverTorque_Fault_trigger"
  Bus Creator/1 -> [EM_Over_temperature_Trigger]  "EM_Over_Temperature_Fault"
  EM_Faulty_Temperature/1 -> Bus Creator/2  "Temp_deg_C"
  Bus Creator1/1 -> [EM_Inverter_Over_temperature_Trigger]  "EM_Inverter_Over_Temperature_Fault"
  EM_Inverter_Faulty_Temperature/1 -> Bus Creator1/2  "Temp_deg_C"
  Trigger1/1 -> Bus Creator1/1  "EM_Inverter_OverTemp_Trigger"
  Bus Creator2/1 -> [EM_Torque_Cmd_Trigger]  "vsm_state_fault"
  EM_torque_cmd_rigger/1 -> Bus Creator2/1  "EM_torque_cmd_trigger"
  EM_torque_cmd_value/1 -> Bus Creator2/2  "EM_torque_cmd_value"

== system EcoSIM3_P2_C2_WIP/Fault Insertion/ESS Triggers ==
  Bus Creator2 : BusCreator  Inputs=3
  Bus Creator3 : BusCreator  Inputs=2
  Chart : Stateflow chart  Commented=on  TreatAsAtomicUnit=on
  ESS_Faulty_Temperature : Constant  Value=0
  ESS_Thermal_Trigger : Constant  Value=0
  Trigger2 : Step  Time=18  After=0  SampleTime=0
  bcm_alarm_trigger : Step  Time=18  After=0  SampleTime=0
  bcm_alarm_type : Constant  Value=0
  tag scope: BCM_Alarm_Trigger=global, ESS_Over_temperature_Trigger=global
  wires:
  Trigger2/1 -> Bus Creator2/1  "ESS_OverTemp_Trigger"
  Bus Creator2/1 -> [ESS_Over_temperature_Trigger]  "ESS_Over_Temperature_Fault"
  ESS_Faulty_Temperature/1 -> Bus Creator2/3  "Temp_deg_C"
  Bus Creator3/1 -> [BCM_Alarm_Trigger]  "bcm_alarm_fault"
  bcm_alarm_trigger/1 -> Bus Creator3/1  "bcm_alarm_trigger"
  bcm_alarm_type/1 -> Bus Creator3/2  "bcm_alarm_type"
  ? -> Chart/1(in)  "ESS_OverTemp_Trigger"
  ESS_Thermal_Trigger/1 -> Bus Creator2/2  "ESS_Thermal_Trigger"

== system EcoSIM3_P2_C2_WIP/GCM/GCM_IO ==
  note: 1) Add Subsystem or Model blocks as valid variant choices.
      | 2) You cannot connect blocks at this level. At simulation, connectivity is automatically
      | determined, based on the active variant and port name matching.
  From_Goto : Subsystem  VariantControl=Sim_type == 1
  VNT Kvaser : Subsystem  VariantControl=Sim_type == 3
  VNT Vector : Subsystem  VariantControl=Sim_type == 2

== system EcoSIM3_P2_C2_WIP/GCM/ProcessMode ==
  note: SWREL12 is the relay signal to power up the remaining softECUs
  note: SWREL11 is the relay signal to power up the MABx, A123, and DCDC
  In1 : Inport
  Bus Creator : BusCreator  Inputs=3
  Bus Creator1 : BusCreator  Inputs=2
  Bus Selector : BusSelector  OutputSignals=GM_Transmit.GM_Electrical_Out.Accessory_Wake,Brusa_Transmit.Brusa_Electrical_Out.GCM_Wakeup_charge
  Chart : Stateflow chart  TreatAsAtomicUnit=on
  MastershiftMessages : Subsystem
  CAN : Outport
  RelaySignals : Outport  Port=2
  wires:
  In1/1 -> MastershiftMessages/1(Inputs), Bus Selector/1
  Bus Creator/1 -> RelaySignals/1
  Bus Selector/1 -> Chart/1(Key_State)  "<Accessory_Wake>"
  Bus Selector/2 -> Chart/2(GCM_Wakeup_charge)  "<GCM_Wakeup_charge>"
  Chart/1(Relay_Charge) -> Bus Creator/1  "Relay_Charge"
  Chart/2(Relay_Vehicle) -> Bus Creator/2  "Relay_Vehicle"
  Chart/3(charge_mode_request) -> Bus Creator1/1  "charge_mode_request"
  Bus Creator1/1 -> CAN/1  "GCM_CAN_Out"
  MastershiftMessages/1(MShift) -> Bus Creator/3
  MastershiftMessages/2(MABx) -> Bus Creator1/2

== system EcoSIM3_P2_C2_WIP/Model Parameters/Cycle Length ==
  Drive Cyc Selection : Inport
  Constant : Constant  Value=inf
  Multiport Switch : MultiPortSwitch  Inputs=10
  Plugged_In : Constant  Value=Veh_Plugged_In
  Switch : Switch  Criteria=u2 > Threshold  Threshold=0.5
  Time : Constant  Value=length(DriveCycles.FUDS.t_cyc)
  Time1 : Constant  Value=length(DriveCycles.FHDS.t_cyc)
  Time2 : Constant  Value=length(DriveCycles.US06.t_cyc)
  Time3 : Constant  Value=length(DriveCycles.Cycle_505.t_cyc)
  Time4 : Constant  Value=length(DriveCycles.US06_City.t_cyc)
  Time5 : Constant  Value=length(DriveCycles.US06_Highway.t_cyc)
  Time6 : Constant  Value=length(DriveCycles.Gradeability.t_cyc)
  Time7 : Constant  Value=length(DriveCycles.Acceleration.t_cyc)
  Time8 : Constant  Value=100
  Time9 : Constant  Value=length(DriveCycles.EC3Y3Fall.t_cyc)
  Cycle Time : Outport
  wires:
  Time/1 -> Multiport Switch/2
  Time1/1 -> Multiport Switch/3
  Time2/1 -> Multiport Switch/4
  Time3/1 -> Multiport Switch/5
  Time4/1 -> Multiport Switch/6
  Time5/1 -> Multiport Switch/7
  Time6/1 -> Multiport Switch/8
  Time7/1 -> Multiport Switch/9
  Drive Cyc Selection/1 -> Multiport Switch/1
  Multiport Switch/1 -> Switch/3
  Time8/1 -> Multiport Switch/10
  Plugged_In/1 -> Switch/2
  Constant/1 -> Switch/1
  Switch/1 -> Cycle Time/1
  Time9/1 -> Multiport Switch/11

== system EcoSIM3_P2_C2_WIP/Model Parameters/Drive Cycle Selection ==
  note: Parameterize-
      | RampSlope
  Drive Cyc Selection : Inport
  505 : simulink/Sources/Repeating Sequence  rep_seq_t=DriveCycles.Cycle_505.t_cyc  rep_seq_y=DriveCycles.Cycle_505.v_cyc
  Acceleration : simulink/Sources/Repeating Sequence  rep_seq_t=DriveCycles.Acceleration.t_cyc  rep_seq_y=DriveCycles.Acceleration.v_cyc
  Acceleration1 : simulink/Sources/Repeating Sequence  rep_seq_t=DriveCycles.EC3Y3Fall.t_cyc  rep_seq_y=DriveCycles.EC3Y3Fall.v_cyc
  Constant : Constant  Value=0
  Demo Cycle : Subsystem
  FHDS : simulink/Sources/Repeating Sequence  rep_seq_t=DriveCycles.FHDS.t_cyc  rep_seq_y=DriveCycles.FHDS.v_cyc
  FUDS : simulink/Sources/Repeating Sequence  rep_seq_t=DriveCycles.FUDS.t_cyc  rep_seq_y=DriveCycles.FUDS.v_cyc
  Gradeability : simulink/Sources/Repeating Sequence  rep_seq_t=DriveCycles.Gradeability.t_cyc  rep_seq_y=DriveCycles.Gradeability.v_cyc
  Multiport Switch : MultiPortSwitch  Inputs=10
  Plugged_In : Constant  Value=Veh_Plugged_In
  Switch : Switch  Criteria=u2 > Threshold  Threshold=0.5
  US06 : simulink/Sources/Repeating Sequence  rep_seq_t=DriveCycles.US06.t_cyc  rep_seq_y=DriveCycles.US06.v_cyc
  US06_City : simulink/Sources/Repeating Sequence  rep_seq_t=DriveCycles.US06_City.t_cyc  rep_seq_y=DriveCycles.US06_City.v_cyc
  US06_Highway : simulink/Sources/Repeating Sequence  rep_seq_t=DriveCycles.US06_Highway.t_cyc  rep_seq_y=DriveCycles.US06_Highway.v_cyc
  Cycle Velocity : Outport
  wires:
  Switch/1 -> Cycle Velocity/1  "Velocity_Profile_m_per_s"
  FUDS/1 -> Multiport Switch/2
  FHDS/1 -> Multiport Switch/3
  US06/1 -> Multiport Switch/4
  505/1 -> Multiport Switch/5
  US06_City/1 -> Multiport Switch/6
  US06_Highway/1 -> Multiport Switch/7
  Gradeability/1 -> Multiport Switch/8
  Acceleration/1 -> Multiport Switch/9
  Drive Cyc Selection/1 -> Multiport Switch/1
  Demo Cycle/1(v) -> Multiport Switch/10
  Multiport Switch/1 -> Switch/3  "Velocity_Profile_m_per_s"
  Plugged_In/1 -> Switch/2
  Constant/1 -> Switch/1
  Acceleration1/1 -> Multiport Switch/11

== system EcoSIM3_P2_C2_WIP/Powertrain/Accessories Power Module ==
  Bus Creator : BusCreator  Inputs=2
  CAN_Receive : Subsystem
  CAN_Transmit : Subsystem
  Component Power : Subsystem
  Plant : Subsystem
  Rate Transition1 : RateTransition
  Subsystem : Subsystem
  Accessories_Power_In_W : Outport
  wires:
  Rate Transition1/1 -> Accessories_Power_In_W/1
  CAN_Receive/1(From_CAN) -> Subsystem/1(CAN_In)
  Plant/1(Sensor_Out) -> Bus Creator/2
  Subsystem/1(To ECU) -> CAN_Transmit/1(To_CAN)
  Subsystem/2(Actuator_Cmds) -> Plant/1(Actuator_Cmds)
  Component Power/1(Out2) -> Bus Creator/1, Rate Transition1/1  "Accessories_Power_In_W"
  Bus Creator/1 -> Subsystem/2(Sensor_In)

== system EcoSIM3_P2_C2_WIP/Powertrain/BAS Motor ==
  note: Power IN or OUT goes to battery????!!
  note: BAS
  " Compnent Model" : Subsystem
  BAS_Receive : Subsystem
  BAS_Transmit : Subsystem
  Soft ECU : Subsystem
  To_Plants : PMIOPort  Port=1  Side=Right
  BAS_Power_in [W] : Outport
  wires:
  " Compnent Model"/2(To_Battery) -> BAS_Power_in [W]/1
  " Compnent Model"/1(Sensor_Out) -> Soft ECU/2(Sensor_In)
  Soft ECU/2(Actuator_Cmds) -> " Compnent Model"/1(Actuator_Cmds)
  Soft ECU/1(CAN_Out) -> BAS_Transmit/1(To_ECUs)
  BAS_Receive/1(From_ECUs) -> Soft ECU/1(CAN_In)
  connections:
  To_Plants/RConn1 -- " Compnent Model"/RConn1

== system EcoSIM3_P2_C2_WIP/Powertrain/Belt Coupler ==
  note: to the BAS
  note: BELT COUPLER
  Belt Drive : sdl_lib/Couplings & Drives/Belt Drive  Commented=on  drive_type=1  belt_type=2  sheave_ang=30 deg  num_belts=8  linear_density=0.6 kg/m  stiffness=1e+4 N/m  damping=1000 N/(m/s)  tension=698 N  breakable=0  F_max=1e+5 N  r_pulley_A=1.1353 in  r_pulley_B=2.8028 in  b_pulley_A=0.001 N*m/(rad/s)  b_pulley_B=0.001 N*m/(rad/s)  model_inertia_A=1  model_inertia_B=1  pulley_inertia_A=0.00001 kg*m^2  pulley_inertia_B=0.00001 kg*m^2  initial_velocity_A=0 rad/s  initial_velocity_B=0 rad/s  mu=0.5  wrap_parameterization=1  d_centers=10.0894 in  phi_wrap_A=145 deg  phi_wrap_B=215 deg  v_thr=0.001 m/s
      settings: LogSimulationData=on
  Sensors : Subsystem
  Simple Gear : sdl_lib/Gears/Simple Gear  ratio=Plants.Belt.GR  rotation_direction=1  friction_model=1  T_noload=0.1 N*m  T_nom=5 N*m  efficiency_nom=0.8  efficiency=0.8  mu_visc=[ 0 0 ] N*m/(rad/s)  w_thr=0.01 rad/s
  BAS Output Shaft1 : PMIOPort  Tag=PMCPort  Port=1  Side=Left
  ICE Output Shaft : PMIOPort  Tag=PMCPort  Port=2  Side=Left
  To_Clutch : PMIOPort  Tag=PMCPort  Port=3  Side=Right
  connections:
  To_Clutch/RConn1 -- Sensors/RConn1
  Simple Gear/LConn1 -- BAS Output Shaft1/RConn1
  Simple Gear/RConn1 -- ICE Output Shaft/RConn1 -- Sensors/LConn1

== system EcoSIM3_P2_C2_WIP/Powertrain/Charger ==
  note: Charger
  Bus Selector : BusSelector  OutputSignals=Veh_Plugged_In
  CAN_Revieve : Subsystem
  CAN_Transmit : Subsystem
  Plant : Subsystem
  Soft ECU : Subsystem
  Charger_Power_W : Outport
  wires:
  [Simulation_Parameters] -> Bus Selector/1
  Bus Selector/1 -> Soft ECU/2(AC)  "<Veh_Plugged_In>"
  CAN_Revieve/1(From_ECUs) -> Soft ECU/1(FromESS)
  Soft ECU/1(ToECUs) -> CAN_Transmit/1(To_CAN)
  Soft ECU/2(Actuator_Cmds) -> Plant/1(FromSoftECU)
  Plant/1(To Plant) -> Charger_Power_W/1

== system EcoSIM3_P2_C2_WIP/Powertrain/Clutch_Transmission1 ==
  note: Transmission
  note: Clutch
  Bus Creator : BusCreator  Inputs=2
  Bus Creator1 : BusCreator  Inputs=2
  Bus Creator2 : BusCreator  Inputs=2
  CAN_Recieve : Subsystem
  CAN_Transmit : Subsystem
  CP1 SoftEcu : Subsystem  Commented=on
  Clutch_Plant : Subsystem
  GCM : Subsystem
  Mastershift Softecu : Subsystem  Commented=on
  Terminator : Terminator
  Trans_Plant : Subsystem
  Shaft : PMIOPort  Tag=PMCPort  Port=1  Side=Left
  Trans Output Shaft : PMIOPort  Port=2  Side=Right
  wires:
  Mastershift Softecu/2(Actuator_Cmds) -> Terminator/1
  GCM/2(To SoftECU) -> CP1 SoftEcu/1(From GCM), Mastershift Softecu/1(From GCM)
  GCM/1(CAN Out) -> CAN_Transmit/1(To_CAN)
  Bus Creator2/1 -> Bus Creator1/2  "Trans_CAN_Out"
  Trans_Plant/2(ActGear) -> Bus Creator2/2
  Bus Creator1/1 -> GCM/2(From CP1)  "SoftECU_Out"
  Mastershift Softecu/1(To_GCM) -> Bus Creator2/1
  CP1 SoftEcu/1(To_GCM) -> Mastershift Softecu/2(Clutch_CAN_Out), Bus Creator1/1
  CAN_Recieve/1(From_CAN) -> GCM/1(CAN_In), Trans_Plant/1(Gear_Cmd), Clutch_Plant/1(Clutch_Engage)
  Bus Creator/1 -> CP1 SoftEcu/2(Sensor_In), Mastershift Softecu/3(Sensor_In)  "Sensor_Out"
  Clutch_Plant/1(Clutch_Status) -> Bus Creator/1
  Trans_Plant/1(Sensor_Out) -> Bus Creator/2
  connections:
  Trans_Plant/RConn1 -- Trans Output Shaft/RConn1
  Clutch_Plant/LConn1 -- Shaft/RConn1
  Clutch_Plant/RConn1 -- Trans_Plant/LConn1

== system EcoSIM3_P2_C2_WIP/Powertrain/Clutch_Transmission2 ==
  note: Clutch
  note: Transmission
  Bus Creator : BusCreator  Inputs=2
  CAN_Recieve : Subsystem
  CAN_Transmit : Subsystem
  CP1 SoftEcu : Subsystem
  Clutch_Plant : Subsystem
  Mastershift Softecu : Subsystem
  Trans_Plant : Subsystem
  Shaft : PMIOPort  Tag=PMCPort  Port=1  Side=Left
  Trans Output Shaft : PMIOPort  Port=2  Side=Right
  wires:
  Trans_Plant/1(Sensor_Out) -> Bus Creator/2
  Clutch_Plant/1(Clutch_Status) -> Bus Creator/1
  Bus Creator/1 -> Mastershift Softecu/2(Sensor_In), CP1 SoftEcu/2(Sensor_In)  "Sensor_Out"
  CP1 SoftEcu/2(Actuator_Cmds) -> Clutch_Plant/1(Clutch_Engage)
  CAN_Recieve/1(From_CAN) -> Mastershift Softecu/1(CANRx), CP1 SoftEcu/1(CANRx)
  CP1 SoftEcu/1(CANTx) -> CAN_Transmit/1(CP1)
  Mastershift Softecu/1(CANTx) -> CAN_Transmit/2(MShift)
  Mastershift Softecu/2(Actuator_Cmds) -> Trans_Plant/1(Gear_Cmd)
  connections:
  Clutch_Plant/RConn1 -- Trans_Plant/LConn1
  Clutch_Plant/LConn1 -- Shaft/RConn1
  Trans_Plant/RConn1 -- Trans Output Shaft/RConn1

== system EcoSIM3_P2_C2_WIP/Powertrain/Electric Motor  ==
  note: Electric Motor
  " Component Model" : Subsystem
  EM_Receive : Subsystem
  EM_Transmit : Subsystem
  Soft ECU : Subsystem
  To_Plants1 : PMIOPort  Port=1  Side=Right
  To_Battery : Outport
  wires:
  " Component Model"/1(Sensor_Out) -> Soft ECU/2(Sensor_In)
  Soft ECU/2(Actuator_Cmds) -> " Component Model"/1(Actuator_Cmds)
  Soft ECU/1(To_ECUs) -> EM_Transmit/1(To_ECUs)
  EM_Receive/1(From_ECUs) -> Soft ECU/1(From_ECUs)
  " Component Model"/2(To_Battery) -> To_Battery/1
  connections:
  " Component Model"/RConn1 -- To_Plants1/RConn1

== system EcoSIM3_P2_C2_WIP/Powertrain/Electrical Storage System ==
  note: ESS
  Charger_Power_In [W] : Inport
  Accessories_Power_In [W] : Inport  Port=2
  EM_Power_In [W] : Inport  Port=3
  BAS_Power_In [W] : Inport  Port=4
  " ESS Model" : Subsystem
  CAN_Revieve : Subsystem
  CAN_Transmit : Subsystem
  Ground : Ground
  Soft ECU : Subsystem
  Terminator : Terminator
  wires:
  " ESS Model"/1(Sensor_Out) -> Soft ECU/2(Sensor_In)
  EM_Power_In [W]/1 -> " ESS Model"/3(EM_Power_In [W])
  Soft ECU/2(Actuator_Cmds) -> " ESS Model"/1(Actuator_Cmds)
  Soft ECU/1(To ECUs) -> CAN_Transmit/1(To_CAN)
  CAN_Revieve/1(From_CAN) -> Soft ECU/1(CAN_In)
  BAS_Power_In [W]/1 -> " ESS Model"/5(BAS_Power_In [W])
  Charger_Power_In [W]/1 -> " ESS Model"/2(Charger_Power_In [W])
  Accessories_Power_In [W]/1 -> Terminator/1
  Ground/1 -> " ESS Model"/4(Accessories_Power_In [W])

== system EcoSIM3_P2_C2_WIP/Powertrain/Engine ==
  note: Engine
  " Component Model" : Subsystem
  ICE_Receive : Subsystem
  ICE_Transmit : Subsystem
  Soft ECU : Subsystem
  ICE Output Shaft : PMIOPort  Tag=PMCPort  Port=1  Side=Right
  Fuel_Consumption : Outport
  wires:
  " Component Model"/1(Sensor_Out) -> Soft ECU/2(Sensor_In)
  Soft ECU/2(Actuator_Cmds) -> " Component Model"/1(Actuator_Cmds)
  Soft ECU/1(ICE_Out) -> ICE_Transmit/1(To_ECUs)
  ICE_Receive/1(From_ECUs) -> Soft ECU/1(ICE_In)
  " Component Model"/2(Fuel_Consumption) -> Fuel_Consumption/1
  connections:
  " Component Model"/RConn1 -- ICE Output Shaft/RConn1

== system EcoSIM3_P2_C2_WIP/Powertrain/Fuel Tank ==
  note: FUEL TANK
  note: This needs to be beta actuator position
  ICE_m_f_dot [kg/s] : Inport
  Add : Sum  Inputs=+-
  Bus Creator1 : BusCreator  Inputs=2
  Divide : Product  Inputs=/*
  Fuel Density : Constant  Value=Plants.ICE.Mdl.Plant.fuel_property.E85_den
  Fuel Density1 : Constant  Value=Plants.Fuel_Tank.Fuel_Cap_Init
  Gain1 : Gain  Gain=1/1000
  Integrator : Integrator
  Terminator : Terminator
  wires:
  Integrator/1 -> Divide/2
  Fuel Density/1 -> Gain1/1
  Divide/1 -> Bus Creator1/2, Add/2  "Fuel_V_f_used_L"
  ICE_m_f_dot [kg/s]/1 -> Integrator/1
  Add/1 -> Bus Creator1/1  "Fuel_Volume_Left_L"
  Bus Creator1/1 -> Terminator/1  "Fuel_Tank_Signals"
  Fuel Density1/1 -> Add/1
  Gain1/1 -> Divide/1

== system EcoSIM3_P2_C2_WIP/Powertrain/Mechanical Coupler ==
  note: MECHANICAL COUPLER
  Inertia2 : fl_lib/Mechanical/Rotational Elements/Inertia  inertia=0.01 kg*m^2  w_specify=off  w_priority=High  w=0 rad/s  t_specify=off  t_priority=High  t=0 N*m
  Sensors : Subsystem
  Simple Gear : sdl_lib/Gears/Simple Gear  ratio=Plants.Mech_Coupler.EM_GR  rotation_direction=1  friction_model=2  T_noload=0.1 N*m  T_nom=5 N*m  efficiency_nom=0.8  efficiency=Plants.Mech_Coupler.EM_Eff  mu_visc=[ 0 0 ] N*m/(rad/s)  w_thr=0.01 rad/s
  EM Output Shaft : PMIOPort  Tag=PMCPort  Port=1  Side=Left
  Trans Output Shaft : PMIOPort  Tag=PMCPort  Port=2  Side=Left
  MC_Coupler_Out : PMIOPort  Tag=PMCPort  Port=3  Side=Right
  connections:
  EM Output Shaft/RConn1 -- Simple Gear/LConn1
  Sensors/LConn1 -- Trans Output Shaft/RConn1 -- Simple Gear/RConn1 -- Inertia2/LConn1
  Sensors/RConn1 -- MC_Coupler_Out/RConn1

== system EcoSIM3_P2_C2_WIP/Powertrain/Soft_ECUs_IO ==
  note: 1) Add Subsystem or Model blocks as valid variant choices.
      | 2) You cannot connect blocks at this level. At simulation, connectivity is automatically
      | determined, based on the active variant and port name matching.
  From_Goto : Subsystem  VariantControl=Sim_type == 1
  VNT Kvaser : Subsystem  VariantControl=Sim_type == 3
  VNT Vector : Subsystem  VariantControl=Sim_type == 2
